simulink model "QC_suspension"  (R2023b)
settings: Solver=VariableStepAuto  StartTime=0.0  StopTime=10.0  RelTol=1e-3
values from neighbouring files (symbols this model uses):
  A = [ ... (first row only)    [QC_params.m]
  B = [ ... (first row only)    [QC_params.m]
  C = [ ... (first row only)    [QC_params.m]
  D = zeros(height(C),width(B))    [QC_params.m]
  IC = zeros(1, 4)    [QC_params.m]    (also in initial_velocity_response.m = scenario.IC)
libraries: simulink x1
settings Model: Creator=joeashton  LastModifiedBy=joeashton

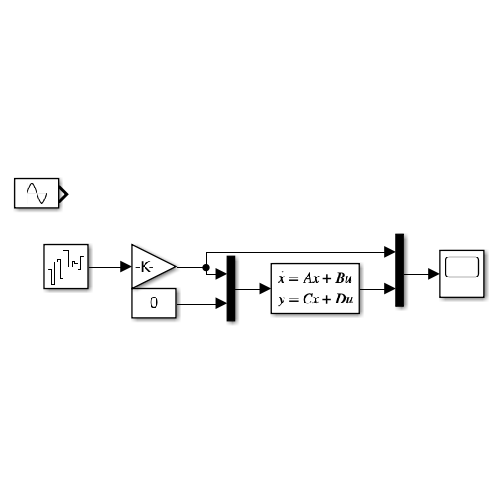
[thumbnail: Simulink's stored preview of the top-level diagram]
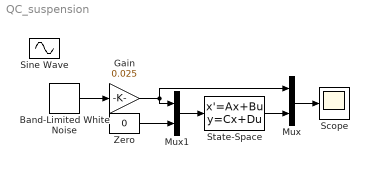
== system QC_suspension ==
  Band-Limited White Noise : simulink/Sources/Band-Limited White Noise  Cov=[0.025]  Ts=0.025  seed=[23341]
  Gain : Gain  Gain=0.025
  Mux : Mux  Inputs=2
  Mux1 : Mux  Inputs=2
  Scope : Scope
  Sine Wave : Sin  Amplitude=0.05  Frequency=100  SampleTime=0
  State-Space : StateSpace  A=A  B=B  C=C  D=D  InitialCondition=IC  ContinuousStateAttributes=['x_b', 'v_b', 'a_b', 'x_w', 'v_b']
  Zero : Constant  Value=0  OutDataTypeStr=Inherit: Inherit via back propagation
  wires:
  Gain/1 -> Mux/1, Mux1/1
  State-Space/1 -> Mux/2
  Mux/1 -> Scope/1
  Mux1/1 -> State-Space/1
  Zero/1 -> Mux1/2
  Band-Limited White Noise/1 -> Gain/1
